simulink model "vehicle_dynamics"  (R2025b)
settings: Solver=FixedStepAuto  StartTime=0.0  StopTime=60  FixedStep=0.005  RelTol=1e-3
libraries: aerolibadyn x1
settings Model: Creator=jWmma  LastModifiedBy=jWmma

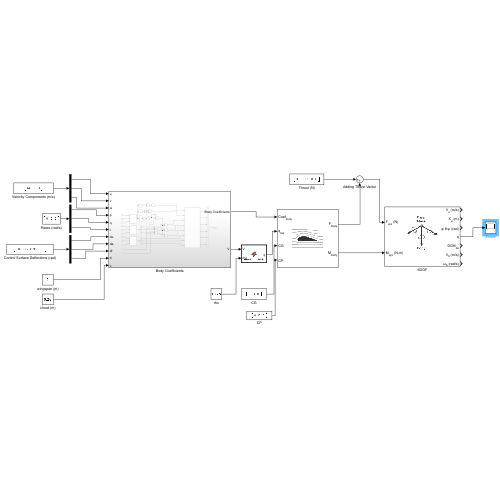
[thumbnail: Simulink's stored preview of the top-level diagram]
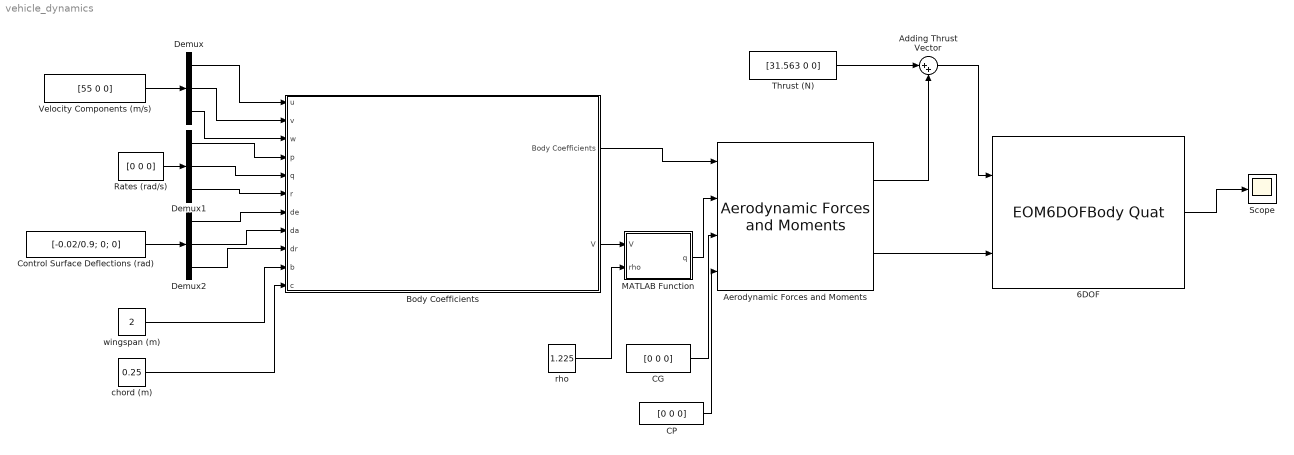
== system vehicle_dynamics ==
  6DOF : EOM6DOFBodyQuat  mass_0=15
  Adding Thrust Vector : Sum  Inputs=|++
  "Aerodynamic Forces and Moments " : aerolibadyn/Aerodynamic Forces and Moments   inputAxes=Body  outputForceAxes=Body  outputMomentAxes=Body  S=0.4  b=2  cbar=0.25
  Body Coefficients : Subsystem
  CG : Constant  Value=[0 0 0]
  CP : Constant  Value=[0 0 0]
  Control Surface Deflections (rad) : Constant  Value=[-0.02/0.9; 0; 0]
  Demux : Demux  Outputs=3
  Demux1 : Demux  Outputs=3
  Demux2 : Demux  Outputs=3
  MATLAB Function : MATLAB Function  TreatAsAtomicUnit=on
  Rates (rad/s) : Constant  Value=[0 0 0]
  Scope : Scope
      settings: ActiveDisplayYMinimum=-29.472290461632362  ActiveDisplayYMaximum=28.031664289649346
  Thrust (N) : Constant  Value=[31.563 0 0]
  Velocity Components (m/s) : Constant  Value=[55 0 0]
  chord (m) : Constant  Value=0.25
  rho : Constant  Value=1.225
  wingspan (m) : Constant  Value=2
  wires:
  Body Coefficients/2(V) -> MATLAB Function/1(V)
  MATLAB Function/1(q) -> "Aerodynamic Forces and Moments "/2
  rho/1 -> MATLAB Function/2(rho)
  Body Coefficients/1(Body Coefficients) -> "Aerodynamic Forces and Moments "/1
  "Aerodynamic Forces and Moments "/1 -> Adding Thrust Vector/2
  CG/1 -> "Aerodynamic Forces and Moments "/3
  CP/1 -> "Aerodynamic Forces and Moments "/4
  wingspan (m)/1 -> Body Coefficients/10(b)
  chord (m)/1 -> Body Coefficients/11(c)
  Control Surface Deflections (rad)/1 -> Demux2/1
  Rates (rad/s)/1 -> Demux1/1
  Velocity Components (m/s)/1 -> Demux/1
  Demux/1 -> Body Coefficients/1(u)
  Demux/2 -> Body Coefficients/2(v)
  Demux/3 -> Body Coefficients/3(w)
  Demux1/1 -> Body Coefficients/4(p)
  Demux1/2 -> Body Coefficients/5(q)
  Demux1/3 -> Body Coefficients/6(r)
  Demux2/1 -> Body Coefficients/7(de)
  Demux2/2 -> Body Coefficients/8(da)
  Demux2/3 -> Body Coefficients/9(dr)
  Thrust (N)/1 -> Adding Thrust Vector/1
  Adding Thrust Vector/1 -> 6DOF/1
  "Aerodynamic Forces and Moments "/2 -> 6DOF/2
  6DOF/4 -> Scope/1

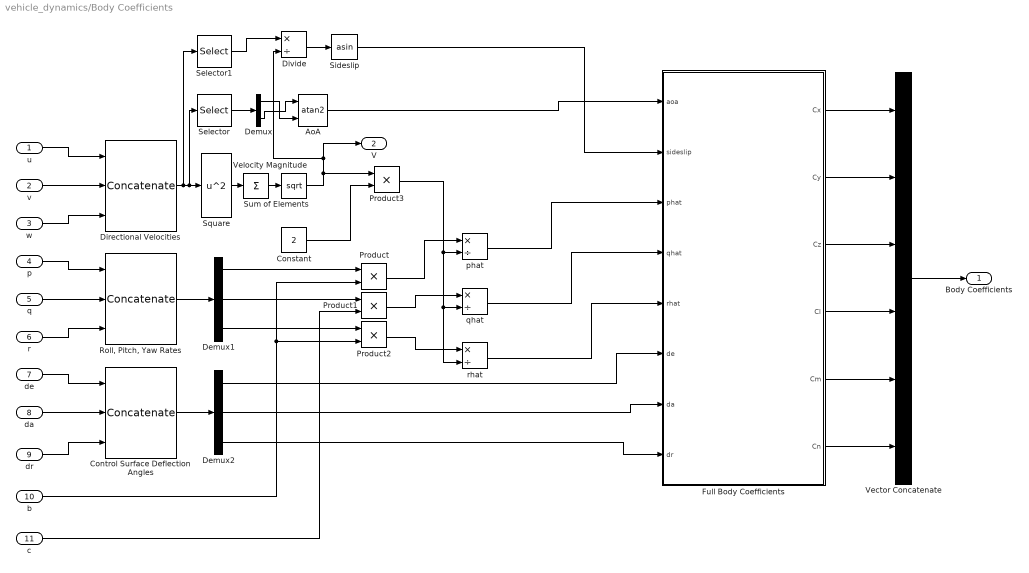
== system vehicle_dynamics/Body Coefficients ==
  u : Inport
  v : Inport  Port=2
  w : Inport  Port=3
  p : Inport  Port=4
  q : Inport  Port=5
  r : Inport  Port=6
  de : Inport  Port=7
  da : Inport  Port=8
  dr : Inport  Port=9
  b : Inport  Port=10
  c : Inport  Port=11
  AoA : Trigonometry  Operator=atan2
  Constant : Constant  Value=2
  Control Surface Deflection Angles : Concatenate  NumInputs=3  ConcatenateDimension=2
  Demux : Demux  Outputs=2
  Demux1 : Demux  Outputs=3
  Demux2 : Demux  Outputs=3
  Directional Velocities : Concatenate  NumInputs=3  ConcatenateDimension=2
  Divide : Product  Inputs=*/
  Full Body Coefficients : MATLAB Function  TreatAsAtomicUnit=on
  Product{,1..3} (4 alike) : Product
  "Roll, Pitch, Yaw Rates" : Concatenate  NumInputs=3  ConcatenateDimension=3
  Selector : Selector  InputPortWidth=3  IndexOptions=Index vector (dialog)  Indices=[1 3]  OutputSizes=1
  Selector1 : Selector  InputPortWidth=3  IndexOptions=Index vector (dialog)  Indices=[2]  OutputSizes=1
  Sideslip : Trigonometry  Operator=asin
  Square : Math  Operator=square
  Sum of Elements : Sum  Inputs=+
  Vector Concatenate : Concatenate  NumInputs=6
  Velocity Magnitude : Sqrt
  phat : Product  Inputs=*/
  qhat : Product  Inputs=*/
  rhat : Product  Inputs=*/
  Body Coefficients : Outport
  V : Outport  Port=2
  wires:
  Demux/2 -> AoA/1
  Selector1/1 -> Divide/1
  b/1 -> Product2/2, Product/2
  Demux1/3 -> Product2/1
  Product2/1 -> rhat/1
  AoA/1 -> Full Body Coefficients/1(aoa)
  Divide/1 -> Sideslip/1
  v/1 -> Directional Velocities/2
  de/1 -> Control Surface Deflection Angles/1
  Velocity Magnitude/1 -> Product3/1, V/1, Divide/2
  Demux2/2 -> Full Body Coefficients/7(da)
  Product/1 -> phat/1
  Directional Velocities/1 -> Selector1/1, Square/1, Selector/1
  Sum of Elements/1 -> Velocity Magnitude/1
  Constant/1 -> Product3/2
  Demux1/1 -> Product/1
  Square/1 -> Sum of Elements/1
  Demux2/1 -> Full Body Coefficients/6(de)
  Sideslip/1 -> Full Body Coefficients/2(sideslip)
  c/1 -> Product1/2
  q/1 -> "Roll, Pitch, Yaw Rates"/2
  Control Surface Deflection Angles/1 -> Demux2/1
  da/1 -> Control Surface Deflection Angles/2
  Demux2/3 -> Full Body Coefficients/8(dr)
  dr/1 -> Control Surface Deflection Angles/3
  Demux1/2 -> Product1/1
  Product3/1 -> phat/2, qhat/2, rhat/2
  w/1 -> Directional Velocities/3
  u/1 -> Directional Velocities/1
  p/1 -> "Roll, Pitch, Yaw Rates"/1
  Selector/1 -> Demux/1
  r/1 -> "Roll, Pitch, Yaw Rates"/3
  rhat/1 -> Full Body Coefficients/5(rhat)
  "Roll, Pitch, Yaw Rates"/1 -> Demux1/1
  phat/1 -> Full Body Coefficients/3(phat)
  qhat/1 -> Full Body Coefficients/4(qhat)
  Product1/1 -> qhat/1
  Vector Concatenate/1 -> Body Coefficients/1
  Demux/1 -> AoA/2
  Full Body Coefficients/1(Cx) -> Vector Concatenate/1
  Full Body Coefficients/2(Cy) -> Vector Concatenate/2
  Full Body Coefficients/3(Cz) -> Vector Concatenate/3
  Full Body Coefficients/4(Cl) -> Vector Concatenate/4
  Full Body Coefficients/5(Cm) -> Vector Concatenate/5
  Full Body Coefficients/6(Cn) -> Vector Concatenate/6

== matlab function vehicle_dynamics/MATLAB Function ==
  data: q output; V input; rho input
function q = dynamic_pressure(V, rho)
q = 1/2 * rho * V^2;
end

== matlab function vehicle_dynamics/Body Coefficients/Full Body Coefficients ==
  data: aoa input; Cx output; sideslip input; phat input; qhat input; rhat input; de input; da input; dr input; Cy output; Cz output; Cl output; Cm output; Cn output
function [Cx,Cy,Cz,Cl,Cm,Cn] = coeffs_body(aoa, sideslip, phat, qhat, rhat, de, da, dr)
%% Coefficients from aerodynamic properties. 
% Change these based on CFD and experimental data

% Lift / Drag / Side force
CL0 = 0.20;    % base lift
CL_a = 5.5;    % lift vs AoA
CL_de = 0.35;  % lift vs elevator
CD0 = 0.04;    % base drag
K = 0.07;      % induced/parasitic drag factor
CY_b = -0.98;  % side force vs sideslip
CY_dr = 0.20;  % side force vs rudder

% Rolling moment
cl_b = -0.12;  % roll vs sideslip
cl_p = -0.55;  % roll damping
cl_r = 0.15;   % roll vs yaw rate
cl_da = 0.10;  % roll vs aileron
cl_dr = 0.02;  % roll vs rudder

% Pitching moment
cm0 = -0.02;  % base pitch
cm_a = -1.20; % pitch vs AoA
cm_q = -12;   % pitch damping
cm_de = -0.90;% pitch vs elevator

% Yawing moment
cn_b = 0.25;  % yaw vs sideslip
cn_p = -0.06; % yaw vs roll rate
cn_r = -0.45; % yaw damping
cn_dr = -0.12;% yaw vs rudder
cn_da= 0.01;  % yaw vs aileron

%% Freestream Coefficients
CL = CL0 + CL_a*aoa + CL_de*de;
CD = CD0 + K*(CL*CL);
CY = CY_b*sideslip + CY_dr*dr;

%% Body Coefficients
Cl = cl_b*sideslip + cl_p*phat + cl_r*rhat + cl_da*da + cl_dr*dr;
Cm = cm0 + cm_a*aoa + cm_q*qhat + cm_de*de;
Cn = cn_b*sideslip + cn_p*phat + cn_r*rhat + cn_dr*dr + cn_da*da;

%% Freestream to Body Rotation
ca=cos(aoa);
sa=sin(aoa);
cb=cos(sideslip);
sb=sin(sideslip);

Xw = -CD;
Yw = CY;
Zw = -CL;

Cx = Xw*ca*cb - Yw*sb + Zw*sa*cb;
Cy = Xw*ca*sb + Yw*cb + Zw*sa*sb;
Cz = -Xw*sa + Zw*ca;

end
